simulink model "GFO_Internal_Forces"  (Simulink 7.5)
settings: Solver=ode45  StartTime=0.0  StopTime=10.0  RelTol=1e-3
undefined symbols (not defined in the file or in its folder): diagmx
libraries: dspmtrx3 x2
settings Model: Creator=konstantinos  LastModifiedBy=konstantinos

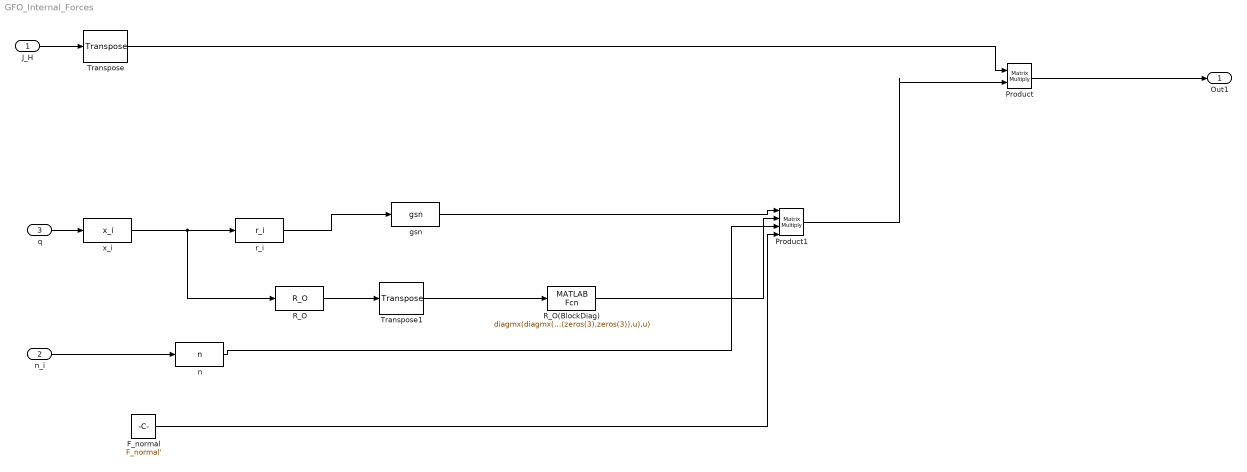
== system GFO_Internal_Forces ==
  J_H : Inport  OutDataType=fixdt(1, 16)  OutScaling=2^0
  n_i : Inport  Port=2  OutDataType=fixdt(1, 16)  OutScaling=2^0
  q : Inport  Port=3  OutDataType=fixdt(1, 16)  OutScaling=2^0
  F_normal : Constant  Value=F_normal'  OutDataType=fixdt(1, 16)  OutScaling=2^0
  Product : Product  Multiplication=Matrix(*)  OutDataType=fixdt(1, 16)  OutScaling=2^0  RndMeth=Zero
  Product1 : Product  Inputs=4  Multiplication=Matrix(*)  OutDataType=fixdt(1, 16)  OutScaling=2^0  RndMeth=Zero
  R_O : MATLABFcn  MATLABFcn=R_O  OutputSignalType=real  Output1D=off
  R_O(BlockDiag) : MATLABFcn  MATLABFcn=diagmx(diagmx(diagmx(zeros(3),zeros(3)),u),u)  OutputSignalType=real  Output1D=off
  Transpose : dspmtrx3/Transpose  SystemSampleTime=-1  Hermitian=off  overflowFlag=off
  Transpose1 : dspmtrx3/Transpose  SystemSampleTime=-1  Hermitian=off  overflowFlag=off
  gsn : MATLABFcn  MATLABFcn=gsn  Output1D=off
  n : MATLABFcn  MATLABFcn=n  Output1D=off
  r_i : MATLABFcn  MATLABFcn=r_i  Output1D=off
  x_i : MATLABFcn  MATLABFcn=x_i  Output1D=off
  Out1 : Outport  OutDataType=fixdt(1, 16)  OutScaling=2^0
  wires:
  Product/1 -> Out1/1
  J_H/1 -> Transpose/1
  Transpose/1 -> Product/1
  q/1 -> x_i/1
  n_i/1 -> n/1
  gsn/1 -> Product1/1
  x_i/1 -> r_i/1, R_O/1
  r_i/1 -> gsn/1
  Product1/1 -> Product/2
  n/1 -> Product1/3
  F_normal/1 -> Product1/4
  R_O(BlockDiag)/1 -> Product1/2
  R_O/1 -> Transpose1/1
  Transpose1/1 -> R_O(BlockDiag)/1
